simulink model "MtrCtrl_24V_2018"  (R2018b)
settings: Solver=FixedStepDiscrete  StartTime=0.0  StopTime=1  FixedStep=1e-6  RelTol=1e-3
values from neighbouring files (symbols this model uses):
  B = 0.001889    [MtrCtrl_v01.sldd]
  C_LUT_AngleTable_sng_Null = 0.0015339807878856412 0.0030679615757712823 0.0046019423636569235 0.0061359231515425647 0.0076699039394282058 0.009203884727313847 0.010737865515199488 0.012271846303085129 0.013805827090970771 0.015339807878856412 0.016873788666742051 0.018407769454627694 0.019941750242513337 0.021475731030398976 0.023009711818284616 0.024543692606170259 0.0260776733940559 0.027611654181941541 0.02914563496982718    [MtrCtrl_v01.sldd]
  C_LUT_SinTable_sng_Null = 0.0015339801862847655 0.0030679567629659761 0.0046019261204485705 0.0061358846491544753 0.007669828739531097 0.00920375478205982 0.010737659167264491 0.012271538285719925 0.013805388528060391 0.0153392062849881 0.01687298794728171 0.01840672990580482 0.019940428551514441 0.021474080275469508 0.023007681468839369 0.024541228522912288 0.0260747178291039 0.02760814577896574 0.029141508764193722 0.030    [MtrCtrl_v01.sldd]
  C_MATH_OneOverSqrtThree_s32n31_Null = 0.57735026918962584    [MtrCtrl_v01.sldd]
  C_MATH_Pi_u32n30_Null = 3.1415926535897931    [MtrCtrl_v01.sldd]
  C_MATH_SqrtThreeOverThree_s32n31_Null = 0.57735026918962573    [MtrCtrl_v01.sldd]
  C_PMSM_CurQKi_u32n31_null = 0.15707963267949    [MtrCtrl_v01.sldd]
  C_PMSM_CurQKp_u32n31_null = 19.949113350295185    [MtrCtrl_v01.sldd]
  C_PMSM_Flux_u32n32_Vs = 0.192    [MtrCtrl_v01.sldd]
  C_PMSM_Ls_pu = 0.398982267005904    [MtrCtrl_v01.sldd]
  C_PMSM_PolePairs_u8_Null = 4.0    [MtrCtrl_v01.sldd]
  Flux = 0.192    [MtrCtrl_v01.sldd]
  IBase_A = 2000.0    [MtrCtrl_v01.sldd]
  J = 0.011    [MtrCtrl_v01.sldd]
  K_CCM_MRASEna_bool_Flg = 0.0    [MtrCtrl_v01.sldd]
  K_SVM_DefultDuty_s32n31_Null = 0.25    [MtrCtrl_v01.sldd]
  KCCM_VirPosn_flg = 0.0    [MtrCtrl_v01.sldd]
  KCCM_VoltModeEna_Flg = 0.0    [MtrCtrl_v01.sldd]
  Kis = 114583.3333333333    [MtrCtrl_v01.sldd]
  KSMO_EnaEst_Flg = 0.0    [MtrCtrl_v01.sldd]
  Kt = 1.1520000000000001    [MtrCtrl_v01.sldd]
  Ld = 0.000635    [MtrCtrl_v01.sldd]
  LPF_coefg = 0.01    [MtrCtrl_v01.sldd]
  Lq = 0.000685    [MtrCtrl_v01.sldd]
  Ls = 0.000635    [MtrCtrl_v01.sldd]
  OneOverUBase_V = 0.0016666666666666668    [MtrCtrl_v01.sldd]
  Pp = 4.0    [MtrCtrl_v01.sldd]
  Rs = 0.05    [MtrCtrl_v01.sldd]
  SecPerRnd = 0.6    [MtrCtrl_v01.sldd]
  SMOGain_V = 323.31615074619043    [MtrCtrl_v01.sldd]
  Ts = 1.0E-6    [MtrCtrl_v01.sldd]
  TsCtrl = 1.0E-6    [MtrCtrl_v01.sldd]
  UBase_V = 600.0    [MtrCtrl_v01.sldd]
  wmBase_rps = 314.15926535897933    [MtrCtrl_v01.sldd]
undefined symbols (not defined in the file or in its folder): DiscIntNeverNeededParam, Ion, Lithium, sinTable
libraries: powerlib x39, simulink x17, ee_lib x16, nesl_utility x6, simulink_extras x2, eePmsmFwController x1, electricdrivelib x1, fl_lib x1
(part 2 of 5)

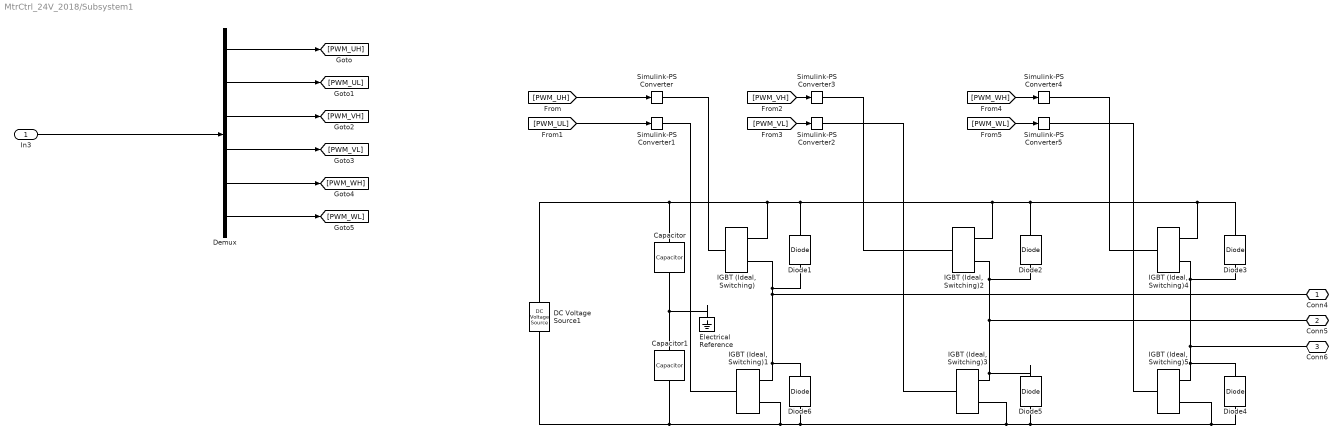
== system MtrCtrl_24V_2018/Subsystem1 ==
  In3 : Inport
  Capacitor : ee_lib/Passive/Capacitor  cap_option=ee.enum.passive.capacitor.capOption.table  c=1e-6 F  Cvec=[0.3125, 6.2500e-02] uF  Vvec=[0, 600] V  CV_table_symmetry=ee.enum.passive.capacitor.tableSymmetry.yes  f_vec=[1, 10] kHz  DFext_vec=[.8, 1.2]  enable_C_tol=ee.enum.toleranceApplication.none  averaging_period=0 s  C_tol=5  tol_distribution=ee.enum.toleranceDistribution.uniform  nSigma=4  r=1e-6 Ohm  g=0 1/Ohm  enable_operating_limits=ee.enum.enable.no  operating_limit_action=ee.enum.passive.reportOpLim.warn  max_working_voltage_range=[-25, 25] V  power_rating=1 W  enable_faults=ee.enum.enable.no  fault_action=simscape.enum.assert.action.none  Cscale_faulted=100  R_faulted=1e-3 Ohm  G_faulted=0 1/Ohm  tau_fault=1e-3 s  fault_trigger=ee.enum.faults.faultTrigger.temporal  t_fault=1 s  max_permissible_voltage_range=[-100, 100] V  t_fail_on_voltage=1 s  i_specify=off  i_priority=None  i=0 A  i_nominal_specify=off  i_nominal_unit=A  i_nominal_value=1  v_specify=off  v_priority=None  v=0 V  v_nominal_specify=off  v_nominal_unit=V  v_nominal_value=1  vc_specify=off  vc_priority=High  vc=0 V  vc_nominal_specify=off  vc_nominal_unit=V  vc_nominal_value=1
  Capacitor1 : ee_lib/Passive/Capacitor  cap_option=ee.enum.passive.capacitor.capOption.table  c=1e-6 F  Cvec=[0.3125, 6.2500e-02] uF  Vvec=[0, 600] V  CV_table_symmetry=ee.enum.passive.capacitor.tableSymmetry.yes  f_vec=[1, 10] kHz  DFext_vec=[.8, 1.2]  enable_C_tol=ee.enum.toleranceApplication.none  averaging_period=0 s  C_tol=5  tol_distribution=ee.enum.toleranceDistribution.uniform  nSigma=4  r=1e-6 Ohm  g=0 1/Ohm  enable_operating_limits=ee.enum.enable.no  operating_limit_action=ee.enum.passive.reportOpLim.warn  max_working_voltage_range=[-25, 25] V  power_rating=1 W  enable_faults=ee.enum.enable.no  fault_action=simscape.enum.assert.action.none  Cscale_faulted=100  R_faulted=1e-3 Ohm  G_faulted=0 1/Ohm  tau_fault=1e-3 s  fault_trigger=ee.enum.faults.faultTrigger.temporal  t_fault=1 s  max_permissible_voltage_range=[-100, 100] V  t_fail_on_voltage=1 s  i_specify=off  i_priority=None  i=0 A  i_nominal_specify=off  i_nominal_unit=A  i_nominal_value=1  v_specify=off  v_priority=None  v=0 V  v_nominal_specify=off  v_nominal_unit=V  v_nominal_value=1  vc_specify=off  vc_priority=High  vc=0 V  vc_nominal_specify=off  vc_nominal_unit=V  vc_nominal_value=1
  DC Voltage Source1 : ee_lib/Additional Components/SPICE Sources/DC Voltage Source  DC=570 V
  Demux : Demux  Outputs=6
  Diode{1..6} (6 alike) : ee_lib/Semiconductors & Converters/Diode  ModelType=ee.enum.diode.modelType.pwl  TableType=ee.enum.diode.tableType.IfMat  IfMat=[.07, .12, .19, 1.75, 4.24, 7.32, 11.2; .16, .3, .72, 2.14, 5.02, 8.35, 13.12] A  VfMat=[.9, 1.15, 1.25, 1.5, 1.75, 2.17, 2.6, 2.85; .58, .68, .75, 1.1, 1.38, 1.77, 2.27, 2.7] V  TjVec=[25, 125] degC  VfVec=[.5, .7, .9, 1.3, 1.7, 2.1, 2.5] V  IfVec=[.1, .2, .5, 1, 2, 4, 7, 10] A  Vf=0.6 V  Ron=0.3 Ohm  Goff=1e-8 S  prmExp=ee.enum.diode.expParam.useTwo  I12=[.0137, .545] A  V12=[.6, .7] V  RS=0 Ohm  Tmeas=25 degC  IS=1e-12 A  ec=1  I1=0.0137 A  V1=0.6 V  N_series=1  N_parallel=1  ZenerEnable=false  Rz=0.3 Ohm  BV=inf V  C_param=ee.enum.diode.capParam.fixed  CJ=0 pF  CJ0=5 pF  Vvec=[.1, 10, 100] V  Cvec=[3.5, 1, .4] pF  VJ=1 V  Mgrad=0.5  FC=0.5  Q_param=ee.enum.diode.recoveryParam.off  iRM=-7.15 A  iF=4 A  didt=-750 A/us  trr_factor=3  trr=115 ns  Qrr=150 nA*s  Vr=-600 V  Ls=150 nH  Erec=0.03 J  TT=50 ns  tau=100 ns  T_param=ee.enum.diode.temperatureParam.off  Tdevice=25 degC  I1_T2=0.245 A  V1_T2=0.5 V  IS_T2=1.25e-7 A  Tmeas2=125 degC  XTI_param=ee.enum.diode.xtiParam.pn  XTI=3  EG_param=ee.enum.diode.egapParam.material_si  EG=1.11 eV  dBVdT=0 V/K  enable_faults=simscape.enum.onoff.off  fault_action=simscape.enum.assert.action.none  fault_types=ee.enum.diode.faults.open  tau_fault=1e-3 s  IfMat_faulted=[.07, .12, .19, 1.75, 4.24, 7.32, 11.2; .16, .3, .72, 2.14, 4.02, 6.35, 9.12] A  VfMat_faulted=[.9, 1.15, 1.25, 1.5, 1.75, 2.17, 2.6, 2.85; .58, .68, .75, 1.1, 1.38, 1.77, 2.27, 2.7] V  VfVec_faulted=[.5, .7, .9, 1.3, 1.7, 2.1, 2.5] V  IfVec_faulted=[.1, .2, .5, 1, 2, 4, 7, 10] A  Ropen_faulted=1000 Ohm  Gshort_faulted=1000 1/Ohm  Vf_faulted=0.6 V  Ron_faulted=0.3 Ohm  Goff_faulted=1e-8 S  I12_faulted=[.0137, .545] A  V12_faulted=[.6, .7] V  IS_faulted=1e-12 A  ec_faulted=1  I1_faulted=0.0137 A  V1_faulted=0.6 V  RS_faulted=0 Ohm  Rz_faulted=0.3 Ohm  BV_faulted=inf V  Cscale_faulted=100  fault_trigger=ee.enum.faults.faultTrigger.temporal  t_fault=inf s  max_permissible_voltage=inf V  n_fail_on_voltage=1  max_permissible_current=inf A  t_fail_on_current=1 s  max_permissible_dVdt=inf V/s  enable_fault_input=simscape.enum.onoff.off  i_specify=off  i_priority=None  i=0 A  i_nominal_specify=off  i_nominal_unit=A  i_nominal_value=1  v_specify=off  v_priority=None  v=0 V  v_nominal_specify=off  v_nominal_unit=V  v_nominal_value=1  v_capacitor_specify=off  v_capacitor_priority=None  v_capacitor=0 V  v_capacitor_nominal_specify=off  v_capacitor_nominal_unit=V  v_capacitor_nominal_value=1  faulted_specify=off  faulted_priority=None  faulted=0  faulted_nominal_specify=off  faulted_nominal_unit=1  faulted_nominal_value=1  i_diode_specify=off  i_diode_priority=None  i_diode=0 A  i_diode_nominal_specify=off  i_diode_nominal_unit=A  i_diode_nominal_value=1  v_diode_specify=off  v_diode_priority=None  v_diode=0 V  v_diode_nominal_specify=off  v_diode_nominal_unit=V  v_diode_nominal_value=1  i_capacitor_specify=off  i_capacitor_priority=None  i_capacitor=0 A  i_capacitor_nominal_specify=off  i_capacitor_nominal_unit=A  i_capacitor_nominal_value=1  power_dissipated_specify=off  power_dissipated_priority=None  power_dissipated=0 W  power_dissipated_nominal_specify=off  power_dissipated_nominal_unit=W  power_dissipated_nominal_value=1  fidelity_level=ee.enum.diode.fidelity.includeChargeDyn  rec_loss_model=ee.enum.diode.reverseRecoveryModel.fixed  ErecVal=0 J  scaleWithIandV=true  ErecMat=zeros(2, 3) J  TjrecVec=[298.15, 398.15] K  IfrecVec=[.1, 1, 10] A  IrecVal=10 A  VrecVal=10 V  tFilter=1 / 1000 / 100 s  max_permissible_temperature=inf K  t_fail_on_temperature=1 s  thermal_network_parameterization=ee.enum.thermalNetworkTopology.junctionCase  Rth=[0, 10] K/W  Rth_Cauer=[1, 3, 10] K/W  Rth_Foster=[4, 6] K/W  thermal_mass_parameterization=ee.enum.thermalNetwork.timeconstant  thermal_mass=[0, 1] J/K  thermal_mass_Cauer=[.1, .3, 1] J/K  thermal_mass_Foster=[1.5, 3] J/K  thermal_time_constant=[0, 10] s  thermal_time_constant_Cauer=[1, 3, 10] s  thermal_time_constant_Foster=[6, 18] s  thermal_mass_initial_temperatures=[25, 25] degC  thermal_mass_initial_temperatures_Cauer=[25, 25, 25] degC  junction_thermal_mass=0.01 J/K  Tvec_initial_Foster=[25, 25, 25, 25] degC  no_thermal_network=0  junction_temperature_specify=off  junction_temperature_priority=None  junction_temperature=25 degC  junction_temperature_nominal_specify=off  junction_temperature_nominal_unit=degC  junction_temperature_nominal_value=1
  Electrical Reference : fl_lib/Electrical/Electrical Elements/Electrical Reference
  IGBT (Ideal, Switching){,1..5} (6 alike) : ee_lib/Semiconductors & Converters/IGBT (Ideal, Switching)  port_option=ee.enum.controlport.ps  Vf=0.8 V  Ron=0.0001 Ohm  Goff=1e-5 1/Ohm  Vth=6 V  diode_param=ee.enum.converters.protectiondiode.none  diode_Vf=0.8 V  diode_Ron=0.001 Ohm  diode_Goff=1e-5 1/Ohm  diode_C=50e-9 F  diode_iRM=-235 A  diode_iF=300 A  diode_idot=-50 A/us  diode_trr_param=ee.enum.converters.diodeReverseParam.trr_factor  diode_trr_factor=3  diode_trr=15 us  diode_Qrr=1500 s*uA  ice_specify=off  ice_priority=None  ice=0 A  ice_nominal_specify=off  ice_nominal_unit=A  ice_nominal_value=1  vce_specify=off  vce_priority=None  vce=0 V  vce_nominal_specify=off  vce_nominal_unit=V  vce_nominal_value=1  vge_specify=off  vge_priority=None  vge=0 V  vge_nominal_specify=off  vge_nominal_unit=V  vge_nominal_value=1  thermal_loss_option=ee.enum.converters.thermalLossOption.constantvalues  Von_data=[0, .1, .6, .8, 1, 1.3, 1.6, 2, 2.4; 0, .1, .7, 1, 1.2, 1.5, 1.9, 2.4, 2.8] V  Tj=[298.15, 398.15] K  Iout_data=[0, .1, 1, 5, 10, 20, 40, 70, 100] A  Eon_data=[0, .0024, .024, .12, .2, .48, 1.04, 2.16, 3.24; 0, .003, .03, .15, .25, .6, 1.3, 2.7, 4.05] * 1e-3 J  Eoff_data=[0, .0007, .0066, .033, .066, .17, .33, .83, 1.5; 0, .001, .01, .05, .1, .25, .5, 1.2, 2.2] * 1e-3 J  Eon_data_3D=[zeros(2, 9, 3)] J  Eoff_data_3D=[zeros(2, 9, 3)] J  Tj_loss=[298.15, 398.15] K  Iout_data_loss=[0, .1, 1, 5, 10, 20, 40, 70, 100] A  tabulateWithVce=false  Vce_loss=[0, 150, 300] V  Eon_scalar=22.86e-3 J  Eoff_scalar=17.14e-3 J  Voff=300 V  Iout_scalar=600 A  useCurrentFromPreviousCycle=false  useVoltageFromPreviousCycle=false  diodeModelType=ee.enum.converters.diodeModelType.pwl  diodeTableType=ee.enum.diode.tableType.IfMat  diode_IfMat=[.07, .12, .19, 1.75, 4.24, 7.32, 11.2; .16, .3, .72, 2.14, 4.02, 6.35, 9.12] A  diode_VfMat=[.9, 1.15, 1.25, 1.5, 1.75, 2.17, 2.6, 2.85; .58, .68, .75, 1.1, 1.38, 1.77, 2.27, 2.7] V  diode_TjVec=[25, 125] degC  diode_VfVec=[.5, .7, .9, 1.3, 1.7, 2.1, 2.5] V  diode_IfVec=[.1, .2, .5, 1, 2, 4, 7, 10] A  diode_Vr=-600 V  diode_Ls=150 nH  diode_Erec=0.03 J  diode_rec_loss_model=ee.enum.diode.reverseRecoveryModel.fixed  diode_ErecVal=0 J  diode_scaleWithIandV=true  diode_ErecMat=zeros(2, 3) J  diode_TjrecVec=[298.15, 398.15] K  diode_IfrecVec=[.1, 1, 10] A  diode_IrecVal=10 A  diode_VrecVal=10 V  diode_tFilter=1 / 1000 / 100 s  thermal_network_parameterization=ee.enum.thermalNetworkTopology.external  Rth=[.08, .5] K/W  Rth_Cauer=[.08, .1, .5] K/W  Rth_Foster=[.08, .14, .22, .16] K/W  thermal_mass_parameterization=ee.enum.thermalNetwork.timeconstant  thermal_mass=[.01, .5] J/K  thermal_mass_Cauer=[.01, .1, .5] J/K  thermal_mass_Foster=[.001, .005, .05, .5] J/K  thermal_time_constant=[.001, .2] s  thermal_time_constant_Cauer=[.001, .1, .2] s  thermal_time_constant_Foster=[7e-05, .0007, .01, .08] s  thermal_mass_initial_temperatures=[25, 25] degC  thermal_mass_initial_temperatures_Cauer=[25, 25, 25] degC  junction_thermal_mass=0.01 J/K  Tvec_initial_Foster=[25, 25, 25, 25] degC  no_thermal_network=0  junction_temperature_specify=off  junction_temperature_priority=None  junction_temperature=25 degC  junction_temperature_nominal_specify=off  junction_temperature_nominal_unit=degC  junction_temperature_nominal_value=1  Qj_specify=off  Qj_priority=None  Qj=0 W  Qj_nominal_specify=off  Qj_nominal_unit=W  Qj_nominal_value=1  accumulatedSwitchingLosses_specify=off  accumulatedSwitchingLosses_priority=None  accumulatedSwitchingLosses=0 J
  Simulink-PS Converter{,1..5} (6 alike) : nesl_utility/Simulink-PS Converter  PhysicalDomain=network_engine_domain  SubClassName=ps_input  LeftPortType=input  RightPortType=output  PseudoPeriodic=off  Frequencies=[]  NoiseDistribution=none  NoiseParameters=[]  Unit=1  AffineConversion=off  FilteringAndDerivatives=provide  SimscapeFilterOrder=1  InputFilterTimeConstant=0.001  UdotUserProvided=0
  Conn4 : PMIOPort  Side=Right
  Conn5 : PMIOPort  Port=2  Side=Right
  Conn6 : PMIOPort  Port=3  Side=Right
  wires:
  [PWM_UL] -> Simulink-PS Converter1/1
  [PWM_UH] -> Simulink-PS Converter/1
  Demux/5 -> [PWM_WH]
  In3/1 -> Demux/1
  Demux/4 -> [PWM_VL]
  Demux/1 -> [PWM_UH]
  Demux/2 -> [PWM_UL]
  Demux/6 -> [PWM_WL]
  Demux/3 -> [PWM_VH]
  [PWM_VH] -> Simulink-PS Converter3/1
  [PWM_VL] -> Simulink-PS Converter2/1
  [PWM_WH] -> Simulink-PS Converter4/1
  [PWM_WL] -> Simulink-PS Converter5/1
  connections:
  "IGBT (Ideal, Switching)5"/RConn1 -- Diode4/RConn1 -- Conn6/RConn1 -- Diode3/LConn1 -- "IGBT (Ideal, Switching)4"/RConn2
  Capacitor/RConn1 -- Capacitor1/LConn1 -- Electrical Reference/LConn1
  Simulink-PS Converter4/RConn1 -- "IGBT (Ideal, Switching)4"/LConn1
  Simulink-PS Converter/RConn1 -- "IGBT (Ideal, Switching)"/LConn1
  "IGBT (Ideal, Switching)"/RConn2 -- Diode6/RConn1 -- "IGBT (Ideal, Switching)1"/RConn1 -- Conn4/RConn1 -- Diode1/LConn1
  Capacitor/LConn1 -- DC Voltage Source1/LConn1 -- Diode3/RConn1 -- "IGBT (Ideal, Switching)4"/RConn1 -- Diode2/RConn1 -- "IGBT (Ideal, Switching)2"/RConn1 -- Diode1/RConn1 -- "IGBT (Ideal, Switching)"/RConn1
  "IGBT (Ideal, Switching)2"/RConn2 -- Diode2/LConn1 -- Diode5/RConn1 -- "IGBT (Ideal, Switching)3"/RConn1 -- Conn5/RConn1
  Diode6/LConn1 -- Capacitor1/RConn1 -- DC Voltage Source1/RConn1 -- "IGBT (Ideal, Switching)1"/RConn2 -- Diode5/LConn1 -- Diode4/LConn1 -- "IGBT (Ideal, Switching)5"/RConn2 -- "IGBT (Ideal, Switching)3"/RConn2
  Simulink-PS Converter3/RConn1 -- "IGBT (Ideal, Switching)2"/LConn1
  "IGBT (Ideal, Switching)5"/LConn1 -- Simulink-PS Converter5/RConn1
  Simulink-PS Converter2/RConn1 -- "IGBT (Ideal, Switching)3"/LConn1
  Simulink-PS Converter1/RConn1 -- "IGBT (Ideal, Switching)1"/LConn1

== system MtrCtrl_24V_2018/Subsystem2 ==
  Bus Creator : BusCreator  Inputs=6
  Bus Creator1 : BusCreator  Inputs=3
  Current Measurement : powerlib/Measurements/Current Measurement  PhasorSimulation=off  OutputType=Complex  PSBequivalent=0
  Current Measurement1 : powerlib/Measurements/Current Measurement  PhasorSimulation=off  OutputType=Complex  PSBequivalent=0
  Current Measurement2 : powerlib/Measurements/Current Measurement  PhasorSimulation=off  OutputType=Complex  PSBequivalent=0
  U : powerlib/Elements/Series RLC Branch  LConnTagsString=__new0  RConnTagsString=__new0  BranchType=RL  Resistance=4.5e-2  Inductance=1.35e-4  SetiL0=off  InitialCurrent=0  Capacitance=1e-6  Setx0=off  InitialVoltage=0  Measurements=None
  V : powerlib/Elements/Series RLC Branch  LConnTagsString=__new0  RConnTagsString=__new0  BranchType=RL  Resistance=4.5e-2  Inductance=1.35e-4  SetiL0=off  InitialCurrent=0  Capacitance=1e-6  Setx0=off  InitialVoltage=0  Measurements=None
  Voltage Measurement{1..6} (6 alike) : powerlib/Measurements/Voltage Measurement  PhasorSimulation=off  OutputType=Complex  PSBequivalent=0
  W : powerlib/Elements/Series RLC Branch  LConnTagsString=__new0  RConnTagsString=__new0  BranchType=RL  Resistance=4.5e-2  Inductance=1.35e-4  SetiL0=off  InitialCurrent=0  Capacitance=1e-6  Setx0=off  InitialVoltage=0  Measurements=None
  A : PMIOPort  Side=Left
  B : PMIOPort  Port=2  Side=Left
  C : PMIOPort  Port=3  Side=Left
  Voltage M : Outport
  Current M : Outport  Port=2
  wires:
  Bus Creator1/1 -> Current M/1
  Current Measurement2/1 -> Bus Creator1/3  "Ic"
  Current Measurement1/1 -> Bus Creator1/2  "Ib"
  Current Measurement/1 -> Bus Creator1/1  "Ia"
  Bus Creator/1 -> Voltage M/1
  Voltage Measurement2/1 -> Bus Creator/4  "Vb"
  Voltage Measurement6/1 -> Bus Creator/6  "Vc"
  Voltage Measurement1/1 -> Bus Creator/5  "Vac"
  Voltage Measurement3/1 -> Bus Creator/1  "Va"
  Voltage Measurement4/1 -> Bus Creator/2  "Vab"
  Voltage Measurement5/1 -> Bus Creator/3  "Vbc"
  connections:
  Current Measurement2/LConn1 -- C/RConn1
  B/RConn1 -- Current Measurement1/LConn1
  Current Measurement/LConn1 -- A/RConn1
  Voltage Measurement4/LConn1 -- Voltage Measurement3/LConn1 -- U/LConn1 -- Current Measurement/RConn1 -- Voltage Measurement1/LConn1
  V/RConn1 -- Voltage Measurement2/LConn2 -- W/RConn1 -- Voltage Measurement6/LConn2 -- Voltage Measurement3/LConn2 -- U/RConn1
  V/LConn1 -- Current Measurement1/RConn1 -- Voltage Measurement2/LConn1 -- Voltage Measurement4/LConn2 -- Voltage Measurement5/LConn1
  W/LConn1 -- Current Measurement2/RConn1 -- Voltage Measurement6/LConn1 -- Voltage Measurement5/LConn2 -- Voltage Measurement1/LConn2

== system MtrCtrl_24V_2018/Subsystem4 ==
  Dlt_Id : Inport
  Dlt_Iq : Inport  Port=2
  we_k : Inport  Port=3
  Dlt_Ud : Inport  Port=4
  Dlt_Uq : Inport  Port=5
  Add{2..5} (4 alike) : Sum
  Constant1 : Constant  Value=0-Ts*Rs/Ls
  Constant14 : Constant  Value=0-Ts*Rs/Ls
  Constant16 : Constant  Value=Ts/Ls
  Constant17 : Constant  Value=Ts/Ls
  Gain6 : Gain  Gain=Ts
  Gain7 : Gain  Gain=-1
  Product{5,9..13} (6 alike) : Product
  Dlt_Id_k1 : Outport
  Dlt_Iq_k1 : Outport  Port=2
  wires:
  Constant17/1 -> Product13/1
  Product10/1 -> Add3/1
  Gain6/1 -> Gain7/1, Product9/2
  Constant1/1 -> Product11/1
  Dlt_Uq/1 -> Product13/2
  Product5/1 -> Add2/1
  Product9/1 -> Add2/2
  Product12/1 -> Add4/2
  Dlt_Id/1 -> Product10/2, Product5/1
  Product11/1 -> Add3/2
  Constant16/1 -> Product12/1
  Add2/1 -> Add4/1
  Dlt_Iq/1 -> Product11/2, Product9/1
  Add5/1 -> Dlt_Iq_k1/1  "Iq_k2"
  we_k/1 -> Gain6/1
  Gain7/1 -> Product10/1
  Constant14/1 -> Product5/2
  Add3/1 -> Add5/1
  Add4/1 -> Dlt_Id_k1/1  "Id_k2"
  Product13/1 -> Add5/2
  Dlt_Ud/1 -> Product12/2

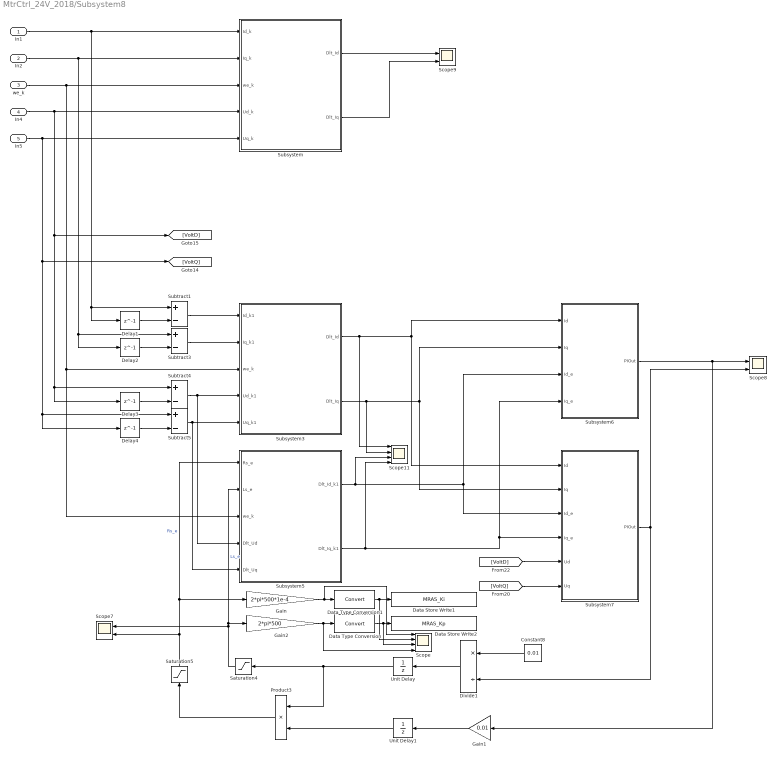
== system MtrCtrl_24V_2018/Subsystem8 ==
  In1 : Inport
  In2 : Inport  Port=2
  we_k : Inport  Port=3
  In4 : Inport  Port=4
  In5 : Inport  Port=5
  Constant8 : Constant  Value=0.01
  Data Store Write1 : DataStoreWrite  DataStoreName=MRAS_Ki
  Data Store Write2 : DataStoreWrite  DataStoreName=MRAS_Kp
  Data Type Conversion : DataTypeConversion
  Data Type Conversion1 : DataTypeConversion
  Delay{1..4} (4 alike) : Delay  DelayLength=1
  Divide1 : Product  Inputs=*/
  Gain : Gain  Gain=2*pi*500*1e-4
  Gain1 : Gain  Gain=0.01
  Gain2 : Gain  Gain=2*pi*500
  Product3 : Product
  Saturation4 : Saturate  UpperLimit=2*Ls  LowerLimit=1e-6
  Saturation5 : Saturate  UpperLimit=1.5*Rs  LowerLimit=1e-6
  Scope : Scope  NumInputPorts=4
  Scope11 : Scope  NumInputPorts=4
  Scope7 : Scope  NumInputPorts=2
  Scope8 : Scope  NumInputPorts=2
  Scope9 : Scope  NumInputPorts=2
  Subsystem : Subsystem
  Subsystem3 : Subsystem
  Subsystem5 : Subsystem
  Subsystem6 : Subsystem
  Subsystem7 : Subsystem
  Subtract{1,3..5} (4 alike) : Sum  Inputs=+-
  Unit Delay : UnitDelay  SampleTime=-1  HasFrameUpgradeWarning=on
  Unit Delay1 : UnitDelay  SampleTime=-1  HasFrameUpgradeWarning=on
  wires:
  Subsystem/1(Dlt_Id) -> Scope9/1
  Delay3/1 -> Subtract4/2
  Subsystem3/1(Dlt_Id) -> Scope11/1, Subsystem6/1(Id), Subsystem7/1(Id)
  Subsystem5/2(Dlt_Iq_k1) -> Scope11/4, Subsystem7/4(Iq_e), Subsystem6/4(Iq_e)
  Subsystem5/1(Dlt_Id_k1) -> Scope11/3, Subsystem6/3(Id_e), Subsystem7/3(Id_e)
  Subsystem6/1(PIOut) -> Scope8/1, Gain1/1
  we_k/1 -> Subsystem5/3(we_k), Subsystem3/3(we_k), Subsystem/3(we_k)
  Subtract4/1 -> Subsystem5/4(Dlt_Ud), Subsystem3/4(Ud_k1)
  Delay1/1 -> Subtract1/2
  [VoltD] -> Subsystem7/5(Ud)
  In5/1 -> [VoltQ], Delay4/1, Subtract5/1, Subsystem/5(Uq_k)
  Subtract5/1 -> Subsystem5/5(Dlt_Uq), Subsystem3/5(Uq_k1)
  In2/1 -> Subtract3/1, Delay2/1, Subsystem/2(Iq_k)
  Subsystem3/2(Dlt_Iq) -> Scope11/2, Subsystem7/2(Iq), Subsystem6/2(Iq)
  Saturation5/1 -> Gain/1, Subsystem5/1(Rs_e), Scope7/2  "Rs_e"
  [VoltQ] -> Subsystem7/6(Uq)
  Constant8/1 -> Divide1/1
  Gain/1 -> Scope/1, Data Type Conversion1/1
  Saturation4/1 -> Gain2/1, Subsystem5/2(Ls_e), Scope7/1  "Ls_e"
  Subtract3/1 -> Subsystem3/2(Iq_k1)
  In1/1 -> Subtract1/1, Delay1/1, Subsystem/1(Id_k)
  Subsystem/2(Dlt_Iq) -> Scope9/2
  Subtract1/1 -> Subsystem3/1(Id_k1)
  Delay4/1 -> Subtract5/2
  Divide1/1 -> Unit Delay/1
  Subsystem7/1(PIOut) -> Divide1/2, Scope8/2
  Unit Delay1/1 -> Product3/2
  Product3/1 -> Saturation5/1
  Delay2/1 -> Subtract3/2
  Unit Delay/1 -> Product3/1, Saturation4/1
  In4/1 -> [VoltD], Delay3/1, Subtract4/1, Subsystem/4(Ud_k)
  Gain2/1 -> Scope/4, Data Type Conversion/1
  Data Type Conversion/1 -> Scope/3, Data Store Write2/1
  Data Type Conversion1/1 -> Scope/2, Data Store Write1/1
  Gain1/1 -> Unit Delay1/1

== system MtrCtrl_24V_2018/TqCtrl ==
  TqRef : Inport
  TqFb : Inport  Port=2
  Sat : Inport  Port=3
  Scope5 : Scope  NumInputPorts=2
  Subsystem1 : Subsystem
  CurSet : Outport
  wires:
  Sat/1 -> Subsystem1/3(Sat)
  TqRef/1 -> Subsystem1/1(Ref), Scope5/1
  TqFb/1 -> Subsystem1/2(Fbk), Scope5/2
  Subsystem1/1(PIOut) -> CurSet/1  "TqPIOut"

== system MtrCtrl_24V_2018/CurLpCtrl/ClarkeTF ==
  CurA : Inport  OutDataTypeStr=fixdt(1,32,31)
  CurB : Inport  Port=2  OutDataTypeStr=fixdt(1,32,31)
  Add : Sum  Inputs=+++  OutDataTypeStr=fixdt(1,32,31)
  Constant : Constant  Value=C_MATH_OneOverSqrtThree_s32n31_Null  OutDataTypeStr=fixdt(1,32,31)
  Data Type Conversion : DataTypeConversion  OutDataTypeStr=fixdt(1,16,15)
  Data Type Conversion1 : DataTypeConversion  OutDataTypeStr=fixdt(1,16,15)
  Data Type Conversion2 : DataTypeConversion
  Product : Product
  I_alpha : Outport
  I_beta : Outport  Port=2
  wires:
  Add/1 -> Data Type Conversion/1
  CurB/1 -> Add/3, Add/2
  CurA/1 -> I_alpha/1, Add/1
  Product/1 -> Data Type Conversion2/1
  Constant/1 -> Data Type Conversion1/1
  Data Type Conversion/1 -> Product/1
  Data Type Conversion1/1 -> Product/2
  Data Type Conversion2/1 -> I_beta/1

== system MtrCtrl_24V_2018/CurLpCtrl/CurCal ==
  CurU : Inport  OutDataTypeStr=fixdt(1,32,31)
  CurW : Inport  Port=2  OutDataTypeStr=fixdt(1,32,31)
  Scope : Scope  NumInputPorts=3
  Subtract : Sum  Inputs=--  OutDataTypeStr=fixdt(1,32,31)
  CurA : Outport
  CurB : Outport  Port=2
  CurC : Outport  Port=3
  wires:
  CurU/1 -> Subtract/1, Scope/1, CurA/1  "Ia"
  CurW/1 -> Subtract/2, Scope/3, CurC/1
  Subtract/1 -> Scope/2, CurB/1  "Ib"

== system MtrCtrl_24V_2018/CurLpCtrl/CurPILp ==
  Id_Ref : Inport  OutDataTypeStr=fixdt(1,32,31)
  Iq_Ref : Inport  Port=2  OutDataTypeStr=fixdt(1,32,31)
  Id_Fb : Inport  Port=3  OutDataTypeStr=fixdt(1,32,31)
  Iq_Fb : Inport  Port=4  OutDataTypeStr=fixdt(1,32,31)
  Udc : Inport  Port=5  OutDataTypeStr=fixdt(0,32,32)
  wm : Inport  Port=6  OutDataTypeStr=fixdt(1,32,31)
  Add : Sum  Inputs=+-  OutDataTypeStr=fixdt(1,32,31)
  Add1 : Sum  OutDataTypeStr=fixdt(1,32,31)
  Constant1 : Constant  Value=KCCM_VoltModeEna_Flg  OutDataTypeStr=boolean
  Constant3 : Constant  Value=100  OutDataTypeStr=fixdt(0,32,25)
  Data Store Read : DataStoreRead  DataStoreName=VoltMode_null
  Display2 : Display
  Display3 : Display
  NOT : Logic  Operator=NOT  AllPortsSameDT=off  OutDataTypeStr=boolean
  OR : Logic  Operator=OR  AllPortsSameDT=off  OutDataTypeStr=boolean
  Scope : Scope  NumInputPorts=3
  Subsystem : Subsystem
  Subsystem1 : Subsystem
  Subsystem2 : Subsystem
  Subsystem3 : Subsystem
  Switch : Switch  Criteria=u2 > Threshold  OutDataTypeStr=fixdt(1,32,32)
  Switch1 : Switch  Criteria=u2 > Threshold  OutDataTypeStr=fixdt(1,32,31)
  Vd : Outport
  Vq : Outport  Port=2
  wires:
  Subsystem1/1(PIOut) -> Switch/1
  Iq_Ref/1 -> Subsystem2/1(Ref)  "IqRef"
  Id_Ref/1 -> Subsystem1/1(Ref)  "IdRef"
  Id_Fb/1 -> Subsystem/2(IdFb), Subsystem1/2(Fbk)  "IdFb"
  Iq_Fb/1 -> Subsystem2/2(Fbk), Subsystem/1(IqFb)  "IqFb"
  OR/1 -> NOT/1
  Switch/1 -> Add/1
  Switch1/1 -> Add1/1
  wm/1 -> Subsystem/3(wm)
  Subsystem/2(Vqff) -> Add1/2, Display2/1  "Vqff"
  Subsystem/1(Vdff) -> Add/2, Display3/1  "Vdff"
  Add1/1 -> Scope/3, Vq/1  "VqCmd"
  Add/1 -> Scope/1, Vd/1  "VdCmd"
  Udc/1 -> Subsystem2/3(Sat), Subsystem1/3(Sat)
  Subsystem2/1(PIOut) -> Switch1/1
  Subsystem3/1(Out1) -> Switch1/3
  Constant3/1 -> Subsystem3/1(Vqcmd)
  Data Store Read/1 -> OR/1
  Constant1/1 -> OR/2
  NOT/1 -> Scope/2, Subsystem/Enable, Switch1/2, Switch/3, Switch/2

== system MtrCtrl_24V_2018/CurLpCtrl/InversePark ==
  D : Inport  OutDataTypeStr=fixdt(1,32,31)
  Q : Inport  Port=2  OutDataTypeStr=fixdt(1,32,31)
  SinTheta : Inport  Port=3  OutDataTypeStr=fixdt(1,32,30)
  CosTheta : Inport  Port=4  OutDataTypeStr=fixdt(1,32,30)
  Scope : Scope  NumInputPorts=2
  dcos : Product  OutDataTypeStr=fixdt(1,32,31)  RndMeth=Simplest
  dsin : Product  OutDataTypeStr=fixdt(1,32,31)  RndMeth=Simplest
  qcos : Product  OutDataTypeStr=fixdt(1,32,31)  RndMeth=Simplest
  qsin : Product  OutDataTypeStr=fixdt(1,32,31)  RndMeth=Simplest
  sum_alpha : Sum  Inputs=|+-  OutDataTypeStr=fixdt(1,32,31)  RndMeth=Simplest
  sum_beta : Sum  Inputs=|++  OutDataTypeStr=fixdt(1,32,31)  RndMeth=Simplest
  Alpha : Outport
  Beta : Outport  Port=2
  wires:
  sum_alpha/1 -> Scope/1, Alpha/1
  sum_beta/1 -> Scope/2, Beta/1
  dsin/1 -> sum_beta/2
  qcos/1 -> sum_beta/1
  CosTheta/1 -> dcos/2, qcos/2
  qsin/1 -> sum_alpha/2
  SinTheta/1 -> qsin/2, dsin/2
  Q/1 -> qcos/1, qsin/1
  dcos/1 -> sum_alpha/1
  D/1 -> dsin/1, dcos/1

== system MtrCtrl_24V_2018/CurLpCtrl/ParkTF ==
  I_alpha : Inport  OutDataTypeStr=fixdt(1,32,31)
  I_beta : Inport  Port=2  OutDataTypeStr=fixdt(1,32,31)
  SinTheta : Inport  Port=3  OutDataTypeStr=fixdt(1,32,30)
  CosTheta : Inport  Port=4  OutDataTypeStr=fixdt(1,32,30)
  Add : Sum  OutDataTypeStr=fixdt(1,32,31)
  Add1 : Sum  Inputs=+-  OutDataTypeStr=fixdt(1,32,31)
  Product{,1..3} (4 alike) : Product  OutDataTypeStr=fixdt(1,32,31)
  Scope : Scope  NumInputPorts=2
  CurD : Outport
  CurQ : Outport  Port=2
  wires:
  Product/1 -> Add/1
  Product1/1 -> Add/2
  Add/1 -> Scope/1, CurD/1
  Add1/1 -> Scope/2, CurQ/1
  Product3/1 -> Add1/1
  Product2/1 -> Add1/2
  I_alpha/1 -> Product2/1, Product/1
  SinTheta/1 -> Product2/2, Product1/2
  I_beta/1 -> Product1/1, Product3/1
  CosTheta/1 -> Product/2, Product3/2

== system MtrCtrl_24V_2018/CurLpCtrl/PhaseCut ==
  In1 : Inport  OutDataTypeStr=fixdt(1,32,4)
  In2 : Inport  Port=2  OutDataTypeStr=fixdt(0,32,33)
  In3 : Inport  Port=3  OutDataTypeStr=fixdt(0,32,33)
  In4 : Inport  Port=4  OutDataTypeStr=fixdt(0,32,33)
  Constant5 : Constant  Value=0.5  OutDataTypeStr=fixdt(0,32,32)
  Constant6 : Constant  Value=0.0  OutDataTypeStr=fixdt(1,32,4)
  Constant7 : Constant  Value=0.00  OutDataTypeStr=fixdt(1,32,4)
  Switch2 : Switch  Criteria=u2 > Threshold  OutDataTypeStr=fixdt(0,32,33)
  Switch3 : Switch  Criteria=u2 > Threshold  OutDataTypeStr=fixdt(0,32,33)
  Switch4 : Switch  Criteria=u2 > Threshold  OutDataTypeStr=fixdt(0,32,33)
  Out1 : Outport
  Out2 : Outport  Port=2
  Out3 : Outport  Port=3
  wires:
  Switch4/1 -> Out3/1
  Constant7/1 -> Switch4/1
  In2/1 -> Switch2/3
  In1/1 -> Switch2/2, Switch3/2, Switch4/2
  Constant5/1 -> Switch2/1
  Switch2/1 -> Out1/1
  Constant6/1 -> Switch3/1
  Switch3/1 -> Out2/1
  In4/1 -> Switch4/3
  In3/1 -> Switch3/3

== system MtrCtrl_24V_2018/CurLpCtrl/SVPWM ==
  Alpha : Inport  OutDataTypeStr=fixdt(1,32,31)
  Beta : Inport  Port=2  OutDataTypeStr=fixdt(1,32,31)
  Add : Sum  OutDataTypeStr=fixdt(0,32,32)
  Gain : Gain  Gain=1/12  OutDataTypeStr=fixdt(0,32,32)
  Overmodulation : Subsystem
  Scope : Scope
  Scope1 : Scope  NumInputPorts=3
  Scope2 : Scope  NumInputPorts=3
  Scope3 : Scope  NumInputPorts=4
  Scope4 : Scope  NumInputPorts=2
  Sector : Subsystem
  SelectRegion : Subsystem  TreatAsAtomicUnit=on
      settings: RTWSystemCode=Nonreusable function  RTWFcnNameOpts=Use subsystem name
  Sn : Subsystem
  Sqrt : Sqrt  OutDataTypeStr=fixdt(0,32,32)  SaturateOnIntegerOverflow=on
  Square : Math  Operator=square  OutDataTypeStr=fixdt(1,32,31)  SaturateOnIntegerOverflow=on
  Square1 : Math  Operator=square  OutDataTypeStr=fixdt(1,32,31)  SaturateOnIntegerOverflow=on
  SwitchTimeCalculation : Subsystem  TreatAsAtomicUnit=on
      settings: RTWSystemCode=Nonreusable function  RTWFcnNameOpts=Use subsystem name
  TempValueCalculation : Subsystem  TreatAsAtomicUnit=on
      settings: RTWSystemCode=Nonreusable function  RTWFcnNameOpts=Use subsystem name
  Sa : Outport
  Sb : Outport  Port=2
  Sc : Outport  Port=3
  wires:
  Sector/2(Tx) -> Overmodulation/1(Tx), Scope4/1
  Overmodulation/1(Tx_out) -> Sn/2(Tx), Scope3/3
  Overmodulation/2(Ty_out) -> Sn/3(Ty), Scope3/4
  Sector/3(Ty) -> Overmodulation/2(Ty), Scope4/2
  Sector/1(Sector) -> Gain/1, Sn/1(Sector), Scope2/3
  Sn/1(Sa) -> Scope3/1, Sa/1
  Sn/2(Sb) -> Sb/1
  Sn/3(Sc) -> Sc/1
  Gain/1 -> Scope3/2
  SelectRegion/1(N) -> SwitchTimeCalculation/1(N)
  TempValueCalculation/3(V3) -> SelectRegion/3(V3), SwitchTimeCalculation/4(V3)  "V2"
  Alpha/1 -> TempValueCalculation/1(V_alpha), Square/1, Scope2/1, Sector/1(Alpha)
  SwitchTimeCalculation/1(Ta) -> Scope1/1  "Ta"
  TempValueCalculation/2(V2) -> SwitchTimeCalculation/3(V2), SelectRegion/2(V2)  "V3"
  TempValueCalculation/1(V1) -> SwitchTimeCalculation/2(V1), SelectRegion/1(V1)  "V1"
  Beta/1 -> Square1/1, Scope2/2, Sector/2(Beta), TempValueCalculation/2(V_beta)
  SwitchTimeCalculation/3(Tc) -> Scope1/3  "Tc"
  SwitchTimeCalculation/2(Tb) -> Scope1/2  "Tb"
  Add/1 -> Sqrt/1
  Square/1 -> Add/1
  Square1/1 -> Add/2
  Sqrt/1 -> Scope/1

== system MtrCtrl_24V_2018/CurLpCtrl/Subsystem10 ==
  idqRef : Inport  OutDataTypeStr=fixdt(1,32,31)
  vdq : Inport  Port=2  OutDataTypeStr=fixdt(1,32,31)
  VphMax : Inport  Port=3  OutDataTypeStr=fixdt(0,32,32)
  PMSM Field-Weakening Controller : eePmsmFwController/PMSM Field-Weakening Controller  Commented=on  Mth=0.95  Kfw=50  Kaw=10  Ts=-1
  Subsystem : Subsystem
  idqRefFW : Outport
  wires:
  vdq/1 -> Subsystem/2(vdq)
  idqRef/1 -> Subsystem/1(idqRef)
  VphMax/1 -> Subsystem/3(VphMax)
  Subsystem/1(idqRefFW) -> idqRefFW/1

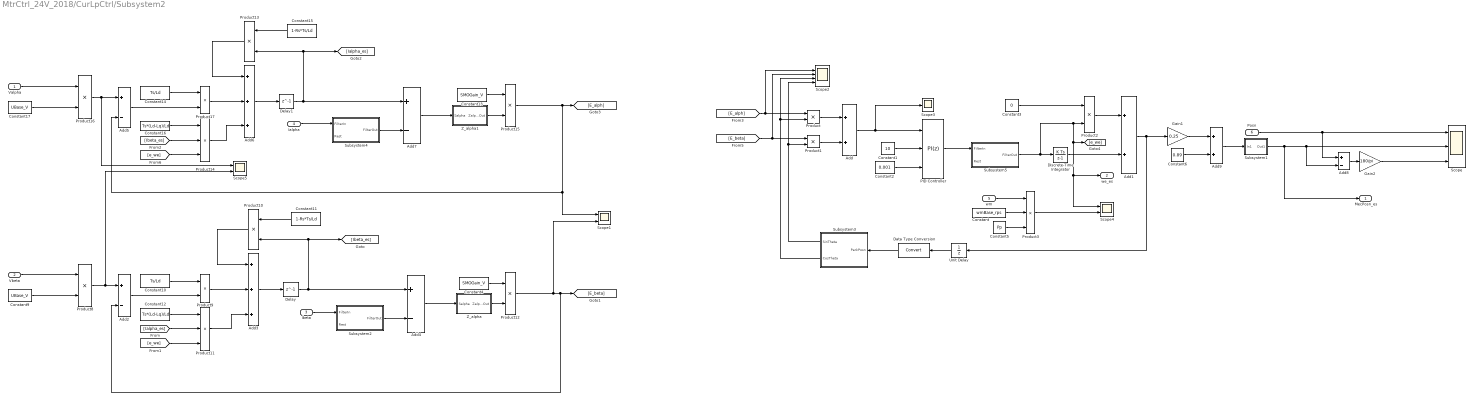
== system MtrCtrl_24V_2018/CurLpCtrl/Subsystem2 ==
  Valpha : Inport  OutDataTypeStr=fixdt(1,32,31)
  Vbeta : Inport  Port=2  OutDataTypeStr=fixdt(1,32,31)
  Ibeta : Inport  Port=3  OutDataTypeStr=fixdt(1,32,31)
  Ialpha : Inport  Port=4  OutDataTypeStr=fixdt(1,32,31)
  wm : Inport  Port=5  OutDataTypeStr=fixdt(1,32,31)
  Posn : Inport  Port=6  OutDataTypeStr=fixdt(1,32,28)
  Add : Sum  OutDataTypeStr=fixdt(1,32,25)
  Add1 : Sum  OutDataTypeStr=fixdt(1,32,24)
  Add2 : Sum  Inputs=+-  OutDataTypeStr=fixdt(1,32,22)
  Add3 : Sum  Inputs=+++  OutDataTypeStr=fixdt(1,32,23)
  Add4 : Sum  Inputs=+-  OutDataTypeStr=int32
  Add5 : Sum  Inputs=+-  OutDataTypeStr=fixdt(1,32,23)
  Add6 : Sum  Inputs=+++  OutDataTypeStr=fixdt(1,32,23)
  Add7 : Sum  Inputs=+-  OutDataTypeStr=fixdt(1,32,0)
  Add8 : Sum  Inputs=+-  OutDataTypeStr=fixdt(1,32,28)
  Add9 : Sum  OutDataTypeStr=fixdt(0,32,0)
  Constant : Constant  Value=wmBase_rps  OutDataTypeStr=fixdt(0,32,23)
  Constant1 : Constant  Value=10  OutDataTypeStr=fixdt(0,32,28)
  Constant10 : Constant  Value=Ts/Ld  OutDataTypeStr=fixdt(0,32,34)
  Constant11 : Constant  Value=1-Rs*Ts/Ld  OutDataTypeStr=fixdt(0,32,32)
  Constant12 : Constant  Value=Ts*(Ld-Lq)/Ld  OutDataTypeStr=fixdt(1,32,47)
  Constant13 : Constant  Value=SMOGain_V  OutDataTypeStr=fixdt(0,32,23)
  Constant14 : Constant  Value=Ts/Ld  OutDataTypeStr=fixdt(0,32,34)
  Constant15 : Constant  Value=1-Rs*Ts/Ld  OutDataTypeStr=fixdt(0,32,32)
  Constant16 : Constant  Value=Ts*(Ld-Lq)/Ld  OutDataTypeStr=fixdt(1,32,47)
  Constant17 : Constant  Value=UBase_V  OutDataTypeStr=fixdt(0,32,22)
  Constant2 : Constant  Value=0.001  OutDataTypeStr=fixdt(0,32,41)
  Constant3 : Constant  Value=0  OutDataTypeStr=fixdt(1,32,4)
  Constant4 : Constant  Value=SMOGain_V  OutDataTypeStr=fixdt(0,32,23)
  Constant5 : Constant  Value=Pp  OutDataTypeStr=fixdt(0,32,29)
  Constant6 : Constant  Value=0.89  OutDataTypeStr=fixdt(0,32,32)
  Constant9 : Constant  Value=UBase_V  OutDataTypeStr=fixdt(0,32,22)
  Data Type Conversion : DataTypeConversion
  Delay : Delay  DelayLength=1
  Delay1 : Delay  DelayLength=1
  Discrete-Time Integrator : DiscreteIntegrator  SampleTime=-1  OutDataTypeStr=fixdt(1,32,24)  ICPrevOutput=DiscIntNeverNeededParam  ICPrevScaledInput=DiscIntNeverNeededParam
  Gain1 : Gain  Gain=0.25  OutDataTypeStr=fixdt(1,32,26)
  Gain2 : Gain  Gain=180/pi  OutDataTypeStr=fixdt(1,32,22)
  PID Controller : simulink/Continuous/PID Controller  Controller=PI  Form=Parallel  TimeDomain=Discrete-time  SampleTime=-1  IntegratorMethod=Forward Euler  ControllerParametersSource=external  P=1  I=1  D=0  N=100  UseFilter=off  TunerSelectOption=Transfer Function Based (PID Tuner App)  InitialConditionSource=internal  InitialConditionForIntegrator=0  InitialConditionForFilter=0  DifferentiatorICPrevScaledInput=0  ExternalReset=none  TrackingMode=off  Kt=1  LimitOutput=off  UpperSaturationLimit=inf  LowerSaturationLimit=-inf  LinearizeAsGain=on  AntiWindupMode=none  Kb=1  PGainOutDataTypeStr=fixdt(1,32,22)  PProdOutDataTypeStr=fixdt(1,32,22)  POutMin=[]  POutMax=[]  IGainOutDataTypeStr=fixdt(1,32,35)  IProdOutDataTypeStr=fixdt(1,32,35)  IOutMin=[]  IOutMax=[]  DOutMin=[]  DOutMax=[]  NOutMin=[]  NOutMax=[]  SumOutDataTypeStr=fixdt(1,32,22)  SumOutMin=[]  SumOutMax=[]  SaturationOutMin=[]  SaturationOutMax=[]  PParamMin=[]  PParamMax=[]  IParamMin=[]  IParamMax=[]  DParamMin=[]  DParamMax=[]  NParamMin=[]  NParamMax=[]  KbParamMin=[]  KbParamMax=[]  KtParamMin=[]  KtParamMax=[]  KbOutMin=[]  KbOutMax=[]  KtOutMin=[]  KtOutMax=[]  IntegratorOutDataTypeStr=fixdt(1,32,24)  IntegratorOutMin=[]  IntegratorOutMax=[]  FilterOutMin=[]  FilterOutMax=[]  SumI1OutMin=[]  SumI1OutMax=[]  SumI2OutMin=[]  SumI2OutMax=[]  SumI3OutMin=[]  SumI3OutMax=[]  SumI4OutMin=[]  SumI4OutMax=[]  SumDOutMin=[]  SumDOutMax=[]  DifferentiatorOutMin=[]  DifferentiatorOutMax=[]  FilterDiffOutCoefMin=[]  FilterDiffOutCoefMax=[]  ReciprocalOutMin=[]  ReciprocalOutMax=[]  SumDenOutMin=[]  SumDenOutMax=[]  SumNumOutMin=[]  SumNumOutMax=[]  DivideOutMin=[]  DivideOutMax=[]  IntegratorContinuousStateAttributes=''  IntegratorStateMustResolveToSignalObject=off  IntegratorRTWStateStorageClass=Auto  FilterContinuousStateAttributes=''  FilterStateMustResolveToSignalObject=off  FilterRTWStateStorageClass=Auto  ParallelPVariant=ExternalParameters  IdealPVariant=Disabled  IVariant=ExternalParameters  DVariant=Disabled  IntegratorVariant=Discrete  SatVariant=Disabled  AWVariant=Passthrough  PCopyVariant=Disabled  TRVariant=Disabled  FdbkBlocksVariant=Forward  IdealPFdbkVariant=Disabled  SatFdbkVariant=Disabled  DerivativeFilterVariant=Disabled  NVariant=Disabled  NCopyVariant=Disabled_SignalSpec  FilterICVariant=Disabled  IntegratorICVariant=InternalICs  ExternalResetVariant=Disabled  TRSumVariant=Passthrough  SumFdbkVariant=Disabled  SumVariant=Sum_PI
  Product{,1,9,12} (4 alike) : Product  OutDataTypeStr=fixdt(1,32,24)
  Product{10,13,15..16} (4 alike) : Product  OutDataTypeStr=fixdt(1,32,23)
  Product11 : Product  Inputs=3  OutDataTypeStr=fixdt(1,32,31)
  Product14 : Product  Inputs=3  OutDataTypeStr=fixdt(1,32,31)
  Product17 : Product  OutDataTypeStr=fixdt(1,32,26)
  Product2 : Product  OutDataTypeStr=fixdt(1,32,4)
  Product3 : Product  Inputs=3  OutDataTypeStr=fixdt(1,32,23)
  Product8 : Product  OutDataTypeStr=fixdt(1,32,22)
  Scope : Scope  NumInputPorts=3
  Scope1 : Scope  NumInputPorts=2
  Scope2 : Scope  NumInputPorts=4
  Scope3 : Scope
  Scope4 : Scope  NumInputPorts=2
  Scope5 : Scope  NumInputPorts=2
  Subsystem1 : Subsystem
  Subsystem2 : Subsystem
  Subsystem3 : Subsystem
  Subsystem4 : Subsystem
  Subsystem5 : Subsystem
  Unit Delay : UnitDelay  SampleTime=-1  HasFrameUpgradeWarning=on
  Z_alpha : Subsystem
  Z_alpha1 : Subsystem
  MecPosn_es : Outport
  we_es : Outport  Port=2
  wires:
  Valpha/1 -> Product16/1
  Constant9/1 -> Product8/2
  Vbeta/1 -> Product8/1
  Add2/1 -> Product9/2
  Constant10/1 -> Product9/1
  Product9/1 -> Add3/2
  Product10/1 -> Add3/1
  Constant11/1 -> Product10/1
  Add3/1 -> Delay/1
  Delay/1 -> Product10/2, [Ibeta_es], Add4/1
  Product11/1 -> Add3/3
  Constant12/1 -> Product11/1
  [Ialpha_es] -> Product11/2
  [e_we] -> Product11/3
  Ibeta/1 -> Subsystem2/1(FilterIn)
  Subsystem2/1(FilterOut) -> Add4/2
  Add4/1 -> Z_alpha/1(Salpha)
  Z_alpha/1(ZalphaOut) -> Product12/2
  Constant4/1 -> Product12/1
  Product12/1 -> Scope1/2, [E_beta], Add2/2
  Product15/1 -> Add5/2, Scope1/1, [E_alph]
  Constant13/1 -> Product15/1
  Z_alpha1/1(ZalphaOut) -> Product15/2
  Add7/1 -> Z_alpha1/1(Salpha)
  Subsystem4/1(FilterOut) -> Add7/2
  [e_we] -> Product14/3
  [Ibeta_es] -> Product14/2
  Constant16/1 -> Product14/1
  Product14/1 -> Add6/3
  Delay1/1 -> Add7/1, [Ialpha_es], Product13/2
  Constant15/1 -> Product13/1
  Product13/1 -> Add6/1
  Product17/1 -> Add6/2
  Constant14/1 -> Product17/1
  Add5/1 -> Product17/2
  Ialpha/1 -> Subsystem4/1(FilterIn)
  Constant17/1 -> Product16/2
  [E_beta] -> Product1/1, Scope2/2
  Product/1 -> Add/1
  Product1/1 -> Add/2
  Add/1 -> PID Controller/1, Scope3/1
  Constant1/1 -> PID Controller/2
  Constant2/1 -> PID Controller/3
  PID Controller/1 -> Subsystem5/1(FilterIn)
  Discrete-Time Integrator/1 -> Add1/2
  Subsystem5/1(FilterOut) -> [e_we], Scope4/1, we_es/1, Product2/2, Discrete-Time Integrator/1
  Constant3/1 -> Product2/1
  Product2/1 -> Add1/1
  Subsystem3/1(SinTheta) -> Product1/2, Scope2/4
  Subsystem3/2(CosTheta) -> Scope2/3, Product/2
  [E_alph] -> Product/1, Scope2/1
  Add8/1 -> Gain2/1
  wm/1 -> Product3/1
  Constant/1 -> Product3/2
  Add1/1 -> Unit Delay/1, Gain1/1
  Constant5/1 -> Product3/3
  Product3/1 -> Scope4/2
  Gain1/1 -> Add9/1
  Constant6/1 -> Add9/2
  Gain2/1 -> Scope/3
  Add9/1 -> Subsystem1/1(In1)
  Posn/1 -> Scope/1, Add8/1
  Subsystem1/1(Out1) -> Scope/2, Add8/2, MecPosn_es/1
  Unit Delay/1 -> Data Type Conversion/1
  Data Type Conversion/1 -> Subsystem3/1(ParkPosn)
  Add6/1 -> Delay1/1
  Product16/1 -> Add5/1, Scope5/1
  Product8/1 -> Scope5/2, Add2/1

== system MtrCtrl_24V_2018/CurLpCtrl/Subsystem4 ==
  IsSet : Inport  OutDataTypeStr=fixdt(1,32,31)
  FluxDegSet : Inport  Port=2  OutDataTypeStr=fixdt(1,32,4)
  Add : Sum  OutDataTypeStr=fixdt(1,32,4)
  Mux : Mux  Inputs=2
  Product : Product  OutDataTypeStr=fixdt(1,32,31)
  Product1 : Product  OutDataTypeStr=fixdt(1,32,31)
  SinCos : Subsystem  Tag=DecoupledSystem
  pi/2 : Constant  Value=0  OutDataTypeStr=fixdt(1,32,4)
  Idq : Outport
  wires:
  SinCos/2(Out2) -> Product1/1
  SinCos/1(Out1) -> Product/2
  IsSet/1 -> Product1/2, Product/1
  FluxDegSet/1 -> Add/1
  Product/1 -> Mux/1
  Product1/1 -> Mux/2
  Add/1 -> SinCos/1(In1)
  pi/2/1 -> Add/2
  Mux/1 -> Idq/1

== system MtrCtrl_24V_2018/CurLpCtrl/Subsystem5 ==
  ParkPosn : Inport  OutDataTypeStr=fixdt(1,32,28)
  1-D Lookup Table : Lookup_n-D  NumberOfTableDimensions=1  BreakpointsForDimension1=C_LUT_AngleTable_sng_Null  BeginIndexSearchUsingPreviousIndexResult=on  Table=C_LUT_SinTable_sng_Null  ExtrapMethod=Clip  UseLastTableValue=on  InternalRulePriority=Speed  OutDataTypeStr=fixdt(0,32,31)  RndMeth=Simplest  InputSameDT=on
  1-D Lookup Table1 : Lookup_n-D  NumberOfTableDimensions=1  BreakpointsForDimension1=C_LUT_AngleTable_sng_Null  BeginIndexSearchUsingPreviousIndexResult=on  Table=C_LUT_SinTable_sng_Null  ExtrapMethod=Clip  UseLastTableValue=on  InternalRulePriority=Speed  OutDataTypeStr=fixdt(0,32,31)  RndMeth=Simplest  InputSameDT=on
  Add : Sum  OutDataTypeStr=fixdt(1,32,26)
  Chart : Stateflow chart  TreatAsAtomicUnit=on
  Constant1 : Constant  Value=0  OutDataTypeStr=fixdt(1,32,4)
  Gain : Gain  Gain=4  OutDataTypeStr=fixdt(1,32,26)
  Product : Product  OutDataTypeStr=fixdt(1,32,30)  RndMeth=Simplest
  Product1 : Product  OutDataTypeStr=fixdt(1,32,30)
  Scope : Scope  NumInputPorts=3
  SinTheta : Outport
  CosTheta : Outport  Port=2
  wires:
  ParkPosn/1 -> Gain/1
  Gain/1 -> Add/2
  Constant1/1 -> Add/1
  Product/1 -> Scope/1, SinTheta/1
  Product1/1 -> Scope/2, CosTheta/1
  Add/1 -> Scope/3, Chart/1(Angle)
  Chart/1(SinAngle) -> 1-D Lookup Table/1
  Chart/3(CosAngle) -> 1-D Lookup Table1/1
  1-D Lookup Table/1 -> Product/1
  Chart/2(SinSign) -> Product/2
  1-D Lookup Table1/1 -> Product1/1
  Chart/4(CosSign) -> Product1/2
